simulink model "x"  (R2016a)
settings: Solver=VariableStepAuto  StartTime=0.0  StopTime=30.0  RelTol=1e-3
settings Model: Creator=Arko  LastModifiedBy=Arko

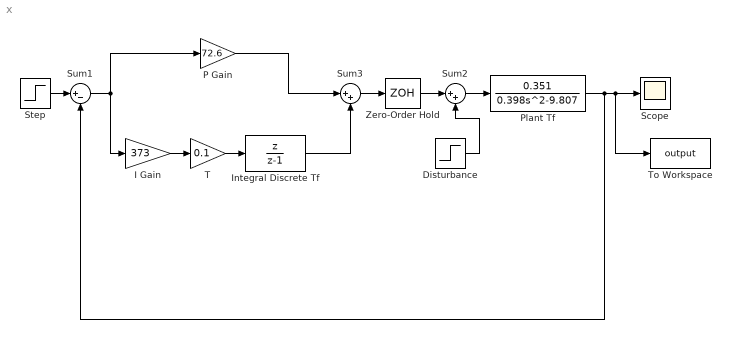
== system x ==
  Disturbance : Step  Time=0  After=0.1  SampleTime=0
  I Gain : Gain  Gain=373
  Integral Discrete Tf : DiscreteTransferFcn  Numerator=[1 0]  Denominator=[1 -1]  SampleTime=0.1
  P Gain : Gain  Gain=72.6
  Plant Tf : TransferFcn  Numerator=[0 0.351]  Denominator="[0.398  0 -9.807]"
  Scope : Scope
  Step : Step  Time=0  SampleTime=0
  Sum1 : Sum  Inputs=|+-
  Sum2 : Sum  Inputs=|++
  Sum3 : Sum  Inputs=|++
  T : Gain  Gain=0.1
  To Workspace : ToWorkspace  VariableName=output  SampleTime=-1
  Zero-Order Hold : ZeroOrderHold  SampleTime=0.1
  wires:
  Step/1 -> Sum1/1
  Plant Tf/1 -> Sum1/2, Scope/1, To Workspace/1
  Sum3/1 -> Zero-Order Hold/1
  I Gain/1 -> T/1
  T/1 -> Integral Discrete Tf/1
  Integral Discrete Tf/1 -> Sum3/2
  P Gain/1 -> Sum3/1
  Sum1/1 -> I Gain/1, P Gain/1
  Zero-Order Hold/1 -> Sum2/1
  Sum2/1 -> Plant Tf/1
  Disturbance/1 -> Sum2/2
